simulink model "q_four_subsys"  (R2019b)
settings: Solver=VariableStepAuto  StartTime=0.0  StopTime=10  RelTol=1e-3
values from neighbouring files (symbols this model uses):
  kq4 = place(A4, B4, p4)    [ex4.m]    (also in ex5.m; ex5test.m)
settings Model: Creator=rafek  LastModifiedBy=rafek

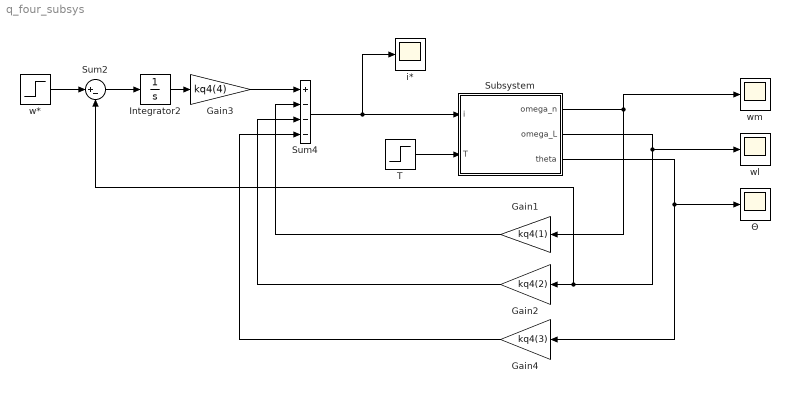
== system q_four_subsys ==
  Gain1 : Gain  Gain=kq4(1)
  Gain2 : Gain  Gain=kq4(2)
  Gain3 : Gain  Gain=kq4(4)
  Gain4 : Gain  Gain=kq4(3)
  Integrator2 : Integrator
  Subsystem : Subsystem
  Sum2 : Sum  Inputs=|+-
  Sum4 : Sum  Inputs=+---
  T : Step  Time=0  After=75  SampleTime=0
  i* : Scope
  w* : Step  Time=0  After=100  SampleTime=0
  wl : Scope
  wm : Scope
  Θ : Scope
  wires:
  Sum2/1 -> Integrator2/1
  Sum4/1 -> i*/1, Subsystem/1(i)
  Gain4/1 -> Sum4/4
  Gain2/1 -> Sum4/3
  Gain3/1 -> Sum4/1
  w*/1 -> Sum2/1
  Subsystem/2(omega_L) -> Sum2/2, Gain2/1, wl/1
  T/1 -> Subsystem/2(T)
  Integrator2/1 -> Gain3/1
  Gain1/1 -> Sum4/2
  Subsystem/3(theta) -> Gain4/1, Θ/1
  Subsystem/1(omega_n) -> wm/1, Gain1/1

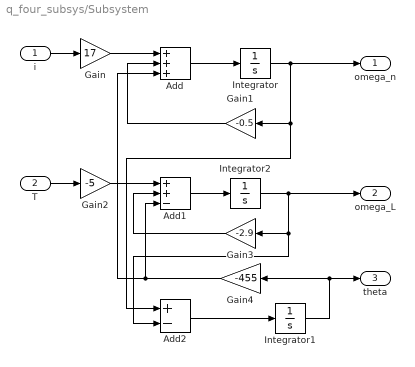
== system q_four_subsys/Subsystem ==
  i : Inport
  T : Inport  Port=2
  Add : Sum  Inputs=+++
  Add1 : Sum  Inputs=++-
  Add2 : Sum  Inputs=+-
  Gain : Gain  Gain=17
  Gain1 : Gain  Gain=-0.5
  Gain2 : Gain  Gain=-5
  Gain3 : Gain  Gain=-2.9
  Gain4 : Gain  Gain=-455
  Integrator : Integrator
  Integrator1 : Integrator
  Integrator2 : Integrator
  omega_n : Outport
  omega_L : Outport  Port=2
  theta : Outport  Port=3
  wires:
  i/1 -> Gain/1
  Gain/1 -> Add/1
  Add/1 -> Integrator/1
  Integrator/1 -> Add2/1, Gain1/1, omega_n/1
  Gain1/1 -> Add/2
  T/1 -> Gain2/1
  Gain2/1 -> Add1/1
  Add2/1 -> Integrator1/1
  Integrator1/1 -> theta/1, Gain4/1
  Gain4/1 -> Add/3, Add1/3
  Gain3/1 -> Add1/2
  Add1/1 -> Integrator2/1
  Integrator2/1 -> Gain3/1, Add2/2, omega_L/1
